simulink model "simu_SPWM"  (R2020b)
settings: Solver=VariableStepAuto  StartTime=0.0  StopTime=0.1  RelTol=1e-3
values from neighbouring files (symbols this model uses):
  G = tf([10*10^9 4.612*10^15 30.342*10^18 15.259*10^-6],[1 561.726*10^3 14.566*10^9 4.918*10^15 33.72*10^18 1.118*10^24])    [Matlab_output_filter.m]
libraries: dspstat3 x2, pid_lib x1, simulink x1
settings Model: Creator=T0264096  LastModifiedBy=T0264096

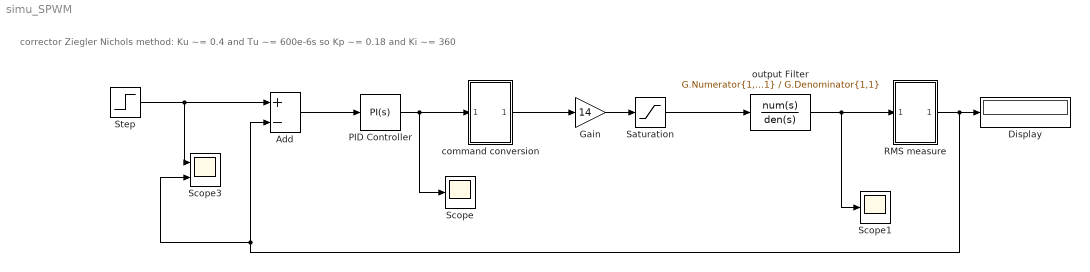
== system simu_SPWM ==
  note: corrector Ziegler Nichols method: Ku ~= 0.4 and Tu ~= 600e-6s so Kp ~= 0.18 and Ki ~= 360
  Add : Sum  Inputs=+-
  Display : Display
  Gain : Gain  Gain=14
  PID Controller : pid_lib/PID Controller  Controller=PI  Form=Parallel  TimeDomain=Continuous-time  UseExternalTs=off  SampleTime=-1  IntegratorMethod=Forward Euler  FilterMethod=Forward Euler  ControllerParametersSource=internal  P=0.22  I=360  D=1.25e-3  UseFilter=on  N=10e10  TunerSelectOption=Transfer Function Based (PID Tuner App)  InitialConditionSource=internal  InitialConditionForIntegrator=0  InitialConditionForFilter=0  DifferentiatorICPrevScaledInput=0  ExternalReset=none  TrackingMode=off  Kt=1  LimitOutput=off  SatLimitsSource=internal  UpperSaturationLimit=inf  LowerSaturationLimit=-inf  LinearizeAsGain=on  AntiWindupMode=none  Kb=1  POutMin=[]  POutMax=[]  IOutMin=[]  IOutMax=[]  DOutMin=[]  DOutMax=[]  NOutMin=[]  NOutMax=[]  SumOutMin=[]  SumOutMax=[]  SaturationOutMin=[]  SaturationOutMax=[]  PParamMin=[]  PParamMax=[]  IParamMin=[]  IParamMax=[]  DParamMin=[]  DParamMax=[]  NParamMin=[]  NParamMax=[]  KbParamMin=[]  KbParamMax=[]  KtParamMin=[]  KtParamMax=[]  KbOutMin=[]  KbOutMax=[]  KtOutMin=[]  KtOutMax=[]  IntegratorOutMin=[]  IntegratorOutMax=[]  FilterOutMin=[]  FilterOutMax=[]  SumI1OutMin=[]  SumI1OutMax=[]  SumI2OutMin=[]  SumI2OutMax=[]  SumI3OutMin=[]  SumI3OutMax=[]  SumI4OutMin=[]  SumI4OutMax=[]  SumDOutMin=[]  SumDOutMax=[]  DifferentiatorOutMin=[]  DifferentiatorOutMax=[]  FilterDiffOutCoefMin=[]  FilterDiffOutCoefMax=[]  ReciprocalOutMin=[]  ReciprocalOutMax=[]  SumDenOutMin=[]  SumDenOutMax=[]  SumNumOutMin=[]  SumNumOutMax=[]  DivideOutMin=[]  DivideOutMax=[]  UdiffTsProdOutMin=[]  UdiffTsProdOutMax=[]  NTsProdOutMin=[]  NTsProdOutMax=[]  UintegralTsProdOutMin=[]  UintegralTsProdOutMax=[]  UngainTsProdOutMin=[]  UngainTsProdOutMax=[]  IntegratorContinuousStateAttributes=''  IntegratorStateMustResolveToSignalObject=off  IntegratorRTWStateStorageClass=Auto  FilterContinuousStateAttributes=''  FilterStateMustResolveToSignalObject=off  FilterRTWStateStorageClass=Auto  ParallelPVariant=InternalParameters  IdealPVariant=Disabled  IVariant=InternalParameters  DVariant=Disabled  IntegratorVariant=Continuous  SatVariant=Disabled  AWVariant=Passthrough  PCopyVariant=Disabled  TRVariant=Disabled  FdbkBlocksVariant=Forward  IdealPFdbkVariant=Disabled  SatFdbkVariant=Disabled  DerivativeFilterVariant=Disabled  NVariant=Disabled  NCopyVariant=Disabled_SignalSpec  FilterICVariant=Disabled  IntegratorICVariant=InternalICs  ExternalResetVariant=Disabled  TRSumVariant=Passthrough  SumFdbkVariant=Disabled  SumVariant=Sum_PI  TsampFilterVariant=InternalTs  TsampNgainVariant=Passthrough  TsampIntegralVariant=Passthrough  ExternalSaturationOutDataTypeStr=Inherit: Same as second input
  RMS measure : Subsystem
  Saturation : Saturate  UpperLimit=14  LowerLimit=0
  Scope : Scope
  Scope1 : Scope
  Scope3 : Scope  NumInputPorts=2
  Step : Step  Time=0.003  After=2  SampleTime=0
  "command conversion " : Subsystem
  output Filter : TransferFcn  Numerator=G.Numerator{1,1}  Denominator=G.Denominator{1,1}
  wires:
  Step/1 -> Add/1, Scope3/1
  RMS measure/1(Out1) -> Display/1, Add/2, Scope3/2
  Add/1 -> PID Controller/1
  "command conversion "/1(Out1) -> Gain/1
  Gain/1 -> Saturation/1
  PID Controller/1 -> Scope/1, "command conversion "/1(In2)
  Saturation/1 -> output Filter/1
  output Filter/1 -> Scope1/1, RMS measure/1(In1)

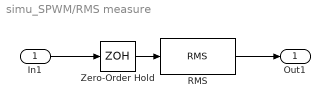
== system simu_SPWM/RMS measure ==
  In1 : Inport
  RMS : dspstat3/RMS  run=on  directionMode=Entire input  dimension=1  reset_popup=None
  Zero-Order Hold : ZeroOrderHold  SampleTime=0.000001
  Out1 : Outport
  wires:
  Zero-Order Hold/1 -> RMS/1
  In1/1 -> Zero-Order Hold/1
  RMS/1 -> Out1/1

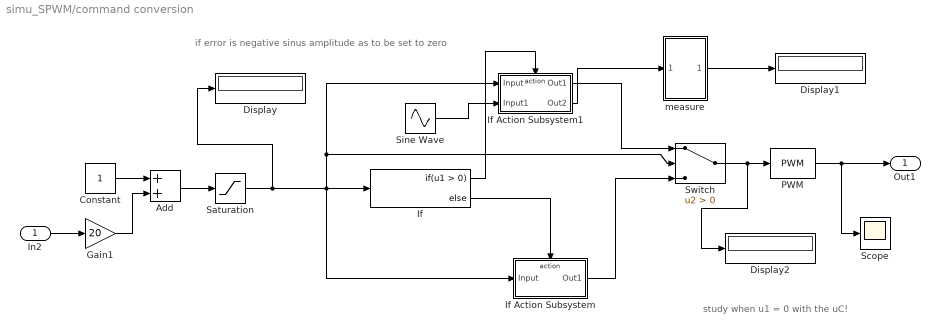
== system simu_SPWM/command conversion  ==
  note: study when u1 = 0 with the uC!
  note: if error is negative sinus amplitude as to be set to zero
  In2 : Inport
  Add : Sum
  Constant : Constant
  Display : Display
  Display1 : Display
  Display2 : Display
  Gain1 : Gain  Gain=20
  If : If
  If Action Subsystem : Subsystem  TreatAsAtomicUnit=on
  If Action Subsystem1 : Subsystem  TreatAsAtomicUnit=on
  PWM : simulink/Discontinuities/PWM  DisableCoverage=on  Period=0.000003  DisallowZeroDutyCycle=off  RunAtFixedTimeIntervals=off  SampleTime=0.1
  Saturation : Saturate  UpperLimit=50  LowerLimit=0
  Scope : Scope
  Sine Wave : Sin  Amplitude=0.4  Frequency=18850  SampleTime=0
  Switch : Switch  Criteria=u2 > Threshold
  measure : Subsystem
  Out1 : Outport
  wires:
  Constant/1 -> Add/1
  In2/1 -> Gain1/1
  Gain1/1 -> Add/2
  Add/1 -> Saturation/1
  Saturation/1 -> Switch/2, If Action Subsystem1/1(Input), If Action Subsystem/1(Input), If/1, Display/1
  If/2 -> If Action Subsystem/Action
  If/1 -> If Action Subsystem1/Action
  If Action Subsystem/1(Out1) -> Switch/3
  If Action Subsystem1/1(Out1) -> Switch/1
  PWM/1 -> Scope/1, Out1/1
  Sine Wave/1 -> If Action Subsystem1/2(Input1)
  If Action Subsystem1/2(Out2) -> measure/1(In1)
  measure/1(Out1) -> Display1/1
  Switch/1 -> Display2/1, PWM/1

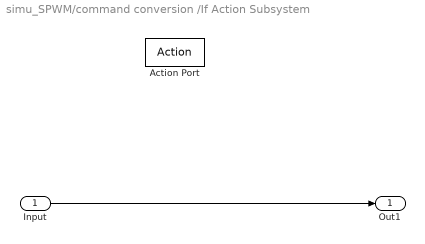
== system simu_SPWM/command conversion /If Action Subsystem ==
  Input : Inport
  Action Port : ActionPort  ActionPortLabel=else
  Out1 : Outport
  wires:
  Input/1 -> Out1/1

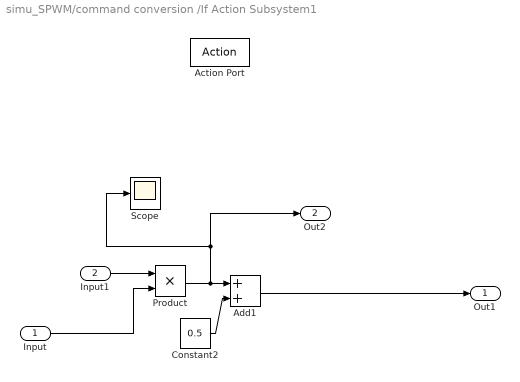
== system simu_SPWM/command conversion /If Action Subsystem1 ==
  Input : Inport
  Input1 : Inport  Port=2
  Action Port : ActionPort  ActionPortLabel=if(u1 > 0)
  Add1 : Sum
  Constant2 : Constant  Value=0.5
  Product : Product
  Scope : Scope
  Out1 : Outport
  Out2 : Outport  Port=2
  wires:
  Constant2/1 -> Add1/2
  Input1/1 -> Product/1
  Product/1 -> Out2/1, Scope/1, Add1/1
  Add1/1 -> Out1/1
  Input/1 -> Product/2

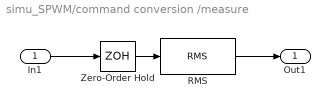
== system simu_SPWM/command conversion /measure ==
  In1 : Inport
  RMS : dspstat3/RMS  run=on  directionMode=Entire input  dimension=1  reset_popup=None
  Zero-Order Hold : ZeroOrderHold  SampleTime=0.000001
  Out1 : Outport
  wires:
  Zero-Order Hold/1 -> RMS/1
  In1/1 -> Zero-Order Hold/1
  RMS/1 -> Out1/1
